simulink model "EZE4sLStEnCtrl"  (R2018b)
settings: Solver=FixedStepDiscrete  StartTime=0.0  StopTime=10.0  FixedStep=0.01  RelTol=1e-3
undefined symbols (not defined in the file or in its folder): data, SecRwLtStBkReclnEn_Clear, SecRwLtStBkReclnEn_Set, SecRwLtStFwdBkwdEn_Clear, SecRwLtStFwdBkwdEn_Set, SecRwLtStHdrstFwdBkwdEn_Clear, SecRwLtStHdrstFwdBkwdEn_Set, SecRwLtStHdrstUpwdDnwdEn_Clear, SecRwLtStHdrstUpwdDnwdEn_Set
libraries: simulink x1
settings Model: Creator=sn2xws  LastModifiedBy=sn55gm
settings DataIOCC: SaveFormat=StructureWithTime
settings OptimizationCC: DefaultParameterBehavior=Inlined  EnhancedBackFolding=on  PassReuseOutputArgsAs=Individual arguments  ZeroExternalMemoryAtStartup=off  ZeroInternalMemoryAtStartup=off  OptimizeBlockOrder=speed  DifferentSizesBufferReuse=on  OptimizationCustomize=off
settings DebuggingCC: ParameterTunabilityLossMsg=error
settings SFSimCC: MATLABDynamicMemAlloc=off
settings RTWCC: SystemTargetFile=autosar.tlc  GenCodeOnly=on  TemplateMakefile=ert_default_tmf  Description=AUTOSAR  GenerateReport=on  IncludeHyperlinkInReport=on  LaunchReport=on  GenerateTraceInfo=on  GenerateTraceReport=on  GenerateTraceReportSl=on  GenerateTraceReportSf=on  GenerateTraceReportEml=on  GenerateCodeMetricsReport=on
settings CodeAppCC: ForceParamTrailComments=on  IgnoreCustomStorageClasses=off  OperatorAnnotations=on  SimulinkDataObjDesc=on  SFDataObjDesc=on  InsertBlockDesc=on
settings STFCustomTargetCC: TargetLangStandard=C99 (ISO)  MultiwordLength=256  ParMdlRefBuildCompliant=on  CompOptLevelCompliant=on  IncludeMdlTerminateFcn=off  CombineOutputUpdateFcns=on  SuppressErrorStatus=on  ERTCustomFileBanners=on  SupportNonFinite=off  SupportComplex=off  SupportContinuousTime=off  SupportNonInlinedSFcns=off  RemoveResetFunc=on  MATLABClassNameForMDSCustomization=Simulink.SoftwareTarget.ERTCustomization  AutosarCompliant=on  UseToolchainInfoCompliant=on  LookupTableObjectStructAxisOrder=2,1,3,4,...  LUTObjectStructOrderEvenSpacing=Size,Table,Breakpoints  SystemTargetFile=autosar.tlc
settings ERTTargetCC: TargetLangStandard=C99 (ISO)  ConcurrentExecutionCompliant=off  IncludeMdlTerminateFcn=off  SuppressErrorStatus=on  SupportNonFinite=off  SupportComplex=off  ModelStepFunctionPrototypeControlCompliant=off  CPPClassGenCompliant=off  AutosarCompliant=on  LookupTableObjectStructAxisOrder=2,1,3,4,...  LUTObjectStructOrderEvenSpacing=Size,Table,Breakpoints  InlinedParameterPlacement=NonHierarchical  ERTCustomFileTemplate=example_file_process.tlc  ERTFilePackagingFormat=Compact

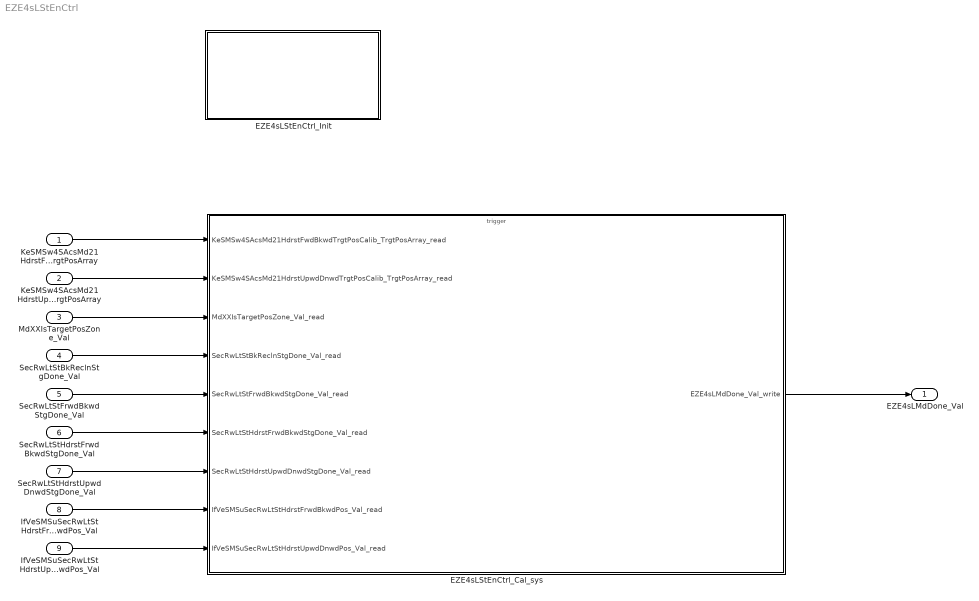
== system EZE4sLStEnCtrl ==
  KeSMSw4SAcsMd21HdrstFwdBkwdTrgtPosCalib_TrgtPosArray : Inport  Description=|  OutDataTypeStr=uint16  PortDimensions=3
      | 0:Pos
      | 1:Max
      | 2:Min
  KeSMSw4SAcsMd21HdrstUpwdDnwdTrgtPosCalib_TrgtPosArray : Inport  Description=|  Port=2  OutDataTypeStr=uint16  PortDimensions=3
      | 0:Pos
      | 1:Max
      | 2:Min
  MdXXIsTargetPosZone_Val : Inport  Port=3  OutDataTypeStr=uint32  PortDimensions=1
  SecRwLtStBkReclnStgDone_Val : Inport  Port=4  OutDataTypeStr=boolean  PortDimensions=1
  SecRwLtStFrwdBkwdStgDone_Val : Inport  Port=5  OutDataTypeStr=boolean  PortDimensions=1
  SecRwLtStHdrstFrwdBkwdStgDone_Val : Inport  Port=6  OutDataTypeStr=boolean  PortDimensions=1
  SecRwLtStHdrstUpwdDnwdStgDone_Val : Inport  Port=7  OutDataTypeStr=boolean  PortDimensions=1
  IfVeSMSuSecRwLtStHdrstFrwdBkwdPos_Val : Inport  Port=8  OutDataTypeStr=uint16  PortDimensions=1
  IfVeSMSuSecRwLtStHdrstUpwdDnwdPos_Val : Inport  Port=9  OutDataTypeStr=uint16  PortDimensions=1
  EZE4sLStEnCtrl_Cal_sys : Subsystem
  EZE4sLStEnCtrl_Init : Subsystem
  EZE4sLMdDone_Val : Outport  OutDataTypeStr=uint8  PortDimensions=1
  wires:
  KeSMSw4SAcsMd21HdrstFwdBkwdTrgtPosCalib_TrgtPosArray/1 -> EZE4sLStEnCtrl_Cal_sys/1(KeSMSw4SAcsMd21HdrstFwdBkwdTrgtPosCalib_TrgtPosArray_read)
  KeSMSw4SAcsMd21HdrstUpwdDnwdTrgtPosCalib_TrgtPosArray/1 -> EZE4sLStEnCtrl_Cal_sys/2(KeSMSw4SAcsMd21HdrstUpwdDnwdTrgtPosCalib_TrgtPosArray_read)
  MdXXIsTargetPosZone_Val/1 -> EZE4sLStEnCtrl_Cal_sys/3(MdXXIsTargetPosZone_Val_read)
  SecRwLtStBkReclnStgDone_Val/1 -> EZE4sLStEnCtrl_Cal_sys/4(SecRwLtStBkReclnStgDone_Val_read)
  SecRwLtStFrwdBkwdStgDone_Val/1 -> EZE4sLStEnCtrl_Cal_sys/5(SecRwLtStFrwdBkwdStgDone_Val_read)
  SecRwLtStHdrstFrwdBkwdStgDone_Val/1 -> EZE4sLStEnCtrl_Cal_sys/6(SecRwLtStHdrstFrwdBkwdStgDone_Val_read)
  SecRwLtStHdrstUpwdDnwdStgDone_Val/1 -> EZE4sLStEnCtrl_Cal_sys/7(SecRwLtStHdrstUpwdDnwdStgDone_Val_read)
  EZE4sLStEnCtrl_Cal_sys/1(EZE4sLMdDone_Val_write) -> EZE4sLMdDone_Val/1
  IfVeSMSuSecRwLtStHdrstFrwdBkwdPos_Val/1 -> EZE4sLStEnCtrl_Cal_sys/8(IfVeSMSuSecRwLtStHdrstFrwdBkwdPos_Val_read)
  IfVeSMSuSecRwLtStHdrstUpwdDnwdPos_Val/1 -> EZE4sLStEnCtrl_Cal_sys/9(IfVeSMSuSecRwLtStHdrstUpwdDnwdPos_Val_read)

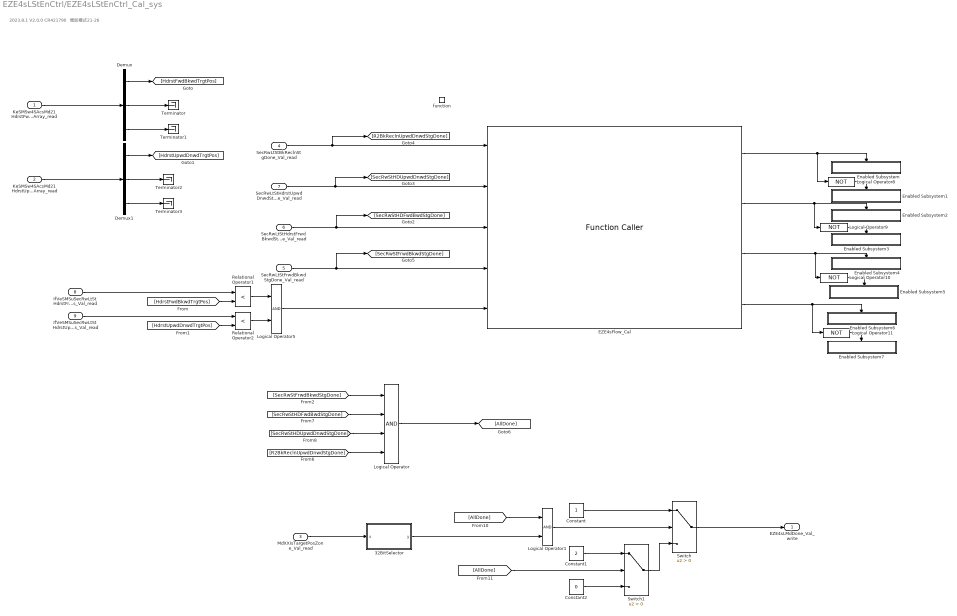
== system EZE4sLStEnCtrl/EZE4sLStEnCtrl_Cal_sys ==
  note: 2023.8.1 V2.0.0 CR421790 增加模式21-26
  KeSMSw4SAcsMd21HdrstFwdBkwdTrgtPosCalib_TrgtPosArray_read : Inport
  KeSMSw4SAcsMd21HdrstUpwdDnwdTrgtPosCalib_TrgtPosArray_read : Inport  Port=2
  MdXXIsTargetPosZone_Val_read : Inport  Port=3
  SecRwLtStBkReclnStgDone_Val_read : Inport  Port=4
  SecRwLtStFrwdBkwdStgDone_Val_read : Inport  Port=5
  SecRwLtStHdrstFrwdBkwdStgDone_Val_read : Inport  Port=6
  SecRwLtStHdrstUpwdDnwdStgDone_Val_read : Inport  Port=7
  IfVeSMSuSecRwLtStHdrstFrwdBkwdPos_Val_read : Inport  Port=8
  IfVeSMSuSecRwLtStHdrstUpwdDnwdPos_Val_read : Inport  Port=9
  function : TriggerPort  TriggerType=function-call  IsSimulinkFunction=on  FunctionName=EZE4sLStEnCtrl_Cal  VariantControl=(inherit)
  32BitSelector : Subsystem  mask(32 Bit Selector){BitNum=20}
      mask prompts: BitNum "Select Bit Number"
      mask help: Allows selection of a particular bit (0-31) out of a packed word up to 32 bits long. Output will be true if the bit number selected via the mask parameter is equal to one.
      mask TypeOptions BitNum: 0 | 1 | 2 | 3 | 4 | 5 | 6 | 7 | 8 | 9 | 10 | 11 | 12 | 13 | 14 | 15 | 16 | 17 | 18 | 19 | 20 | 21 | 22 | 23 | 24 | 25 | 26 | 27 | 28 | 29 | 30 | 31
      mask Display:
      | text(0.5, 0.8,'BIT','horizontalAlignment','center')
      | text(0.5, 0.5,'SELECTOR','horizontalAlignment','center')
      | text(0.5, 0.2,['-- Bit ',char(get_param(gcb,'BitNum')),' --'],'horizontalAlignment','center')
  Constant : Constant  OutDataTypeStr=uint8
  Constant1 : Constant  Value=2  OutDataTypeStr=uint8
  Constant2 : Constant  Value=0  OutDataTypeStr=uint8
  Demux : Demux  Outputs=3
  Demux1 : Demux  Outputs=3
  EZE4sFlow_Cal : FunctionCaller  FunctionPrototype=[BkReclnEn,HdrstUpwdEn,HdrstFrwdEn,SecRwStFrwdBkwdEn] = EZE4sFlow_Cal(BkReclnStgDone,HdrstUpwdDnwdStgDone,HdrstFrwdBkwdStgDone,SecRwStFrwdBkwdStgDone,Chkhdflg)  InputArgumentSpecifications=boolean(true), boolean(true), boolean(true), boolean(true), boolean(true)  OutputArgumentSpecifications=boolean(true), boolean(true), boolean(true), boolean(true)
  Enabled Subsystem : Subsystem  TreatAsAtomicUnit=on
  Enabled Subsystem1 : Subsystem  TreatAsAtomicUnit=on
  Enabled Subsystem2 : Subsystem  TreatAsAtomicUnit=on
  Enabled Subsystem3 : Subsystem  TreatAsAtomicUnit=on
  Enabled Subsystem4 : Subsystem  TreatAsAtomicUnit=on
  Enabled Subsystem5 : Subsystem  TreatAsAtomicUnit=on
  Enabled Subsystem6 : Subsystem  TreatAsAtomicUnit=on
  Enabled Subsystem7 : Subsystem  TreatAsAtomicUnit=on
  Logical Operator : Logic  Inputs=4  AllPortsSameDT=off  OutDataTypeStr=boolean
  Logical Operator1 : Logic  AllPortsSameDT=off  OutDataTypeStr=boolean
  Logical Operator{8..11} (4 alike) : Logic  Operator=NOT  AllPortsSameDT=off  OutDataTypeStr=boolean
  Logical Operator5 : Logic  AllPortsSameDT=off  OutDataTypeStr=boolean
  Relational Operator1 : RelationalOperator  Operator=<  OutDataTypeStr=boolean  RndMeth=Simplest
  Relational Operator2 : RelationalOperator  Operator=<  OutDataTypeStr=boolean  RndMeth=Simplest
  Switch : Switch  Criteria=u2 > Threshold
  Switch1 : Switch  Criteria=u2 > Threshold
  Terminator{,1..3} (4 alike) : Terminator
  EZE4sLMdDone_Val_write : Outport
      settings: EnsureOutportIsVirtual=on
  wires:
  Relational Operator1/1 -> Logical Operator5/1
  Logical Operator5/1 -> EZE4sFlow_Cal/5
  Relational Operator2/1 -> Logical Operator5/2
  SecRwLtStBkReclnStgDone_Val_read/1 -> [R2BkReclnUpwdDnwdStgDone], EZE4sFlow_Cal/1
  SecRwLtStHdrstUpwdDnwdStgDone_Val_read/1 -> [SecRwStHDUpwdDnwdStgDone], EZE4sFlow_Cal/2
  SecRwLtStFrwdBkwdStgDone_Val_read/1 -> [SecRwStFrwdBkwdStgDone], EZE4sFlow_Cal/4
  SecRwLtStHdrstFrwdBkwdStgDone_Val_read/1 -> [SecRwStHDFwdBwdStgDone], EZE4sFlow_Cal/3
  IfVeSMSuSecRwLtStHdrstFrwdBkwdPos_Val_read/1 -> Relational Operator1/1
  IfVeSMSuSecRwLtStHdrstUpwdDnwdPos_Val_read/1 -> Relational Operator2/1
  KeSMSw4SAcsMd21HdrstFwdBkwdTrgtPosCalib_TrgtPosArray_read/1 -> Demux/1
  Demux/1 -> [HdrstFwdBkwdTrgtPos]
  KeSMSw4SAcsMd21HdrstUpwdDnwdTrgtPosCalib_TrgtPosArray_read/1 -> Demux1/1
  Demux1/1 -> [HdrstUpwdDnwdTrgtPos]
  Demux/2 -> Terminator/1
  Demux/3 -> Terminator1/1
  Demux1/2 -> Terminator2/1
  Demux1/3 -> Terminator3/1
  [HdrstFwdBkwdTrgtPos] -> Relational Operator1/2
  [HdrstUpwdDnwdTrgtPos] -> Relational Operator2/2
  [SecRwStHDUpwdDnwdStgDone] -> Logical Operator/3
  [SecRwStHDFwdBwdStgDone] -> Logical Operator/2
  [R2BkReclnUpwdDnwdStgDone] -> Logical Operator/4
  [SecRwStFrwdBkwdStgDone] -> Logical Operator/1
  Constant1/1 -> Switch1/1
  Constant/1 -> Switch/1
  Switch1/1 -> Switch/3
  Logical Operator1/1 -> Switch/2
  [AllDone] -> Logical Operator1/1
  32BitSelector/1(y) -> Logical Operator1/2
  Switch/1 -> EZE4sLMdDone_Val_write/1
  [AllDone] -> Switch1/2
  MdXXIsTargetPosZone_Val_read/1 -> 32BitSelector/1(x)
  Constant2/1 -> Switch1/3
  Logical Operator/1 -> [AllDone]
  EZE4sFlow_Cal/2 -> Logical Operator9/1, Enabled Subsystem2/Enable
  Logical Operator10/1 -> Enabled Subsystem5/Enable
  Logical Operator8/1 -> Enabled Subsystem1/Enable
  EZE4sFlow_Cal/3 -> Logical Operator10/1, Enabled Subsystem4/Enable
  EZE4sFlow_Cal/1 -> Logical Operator8/1, Enabled Subsystem/Enable
  Logical Operator9/1 -> Enabled Subsystem3/Enable
  Logical Operator11/1 -> Enabled Subsystem7/Enable
  EZE4sFlow_Cal/4 -> Logical Operator11/1, Enabled Subsystem6/Enable

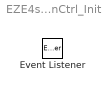
== system EZE4sLStEnCtrl/EZE4sLStEnCtrl_Init ==
  Event Listener : EventListener  EventName=reset

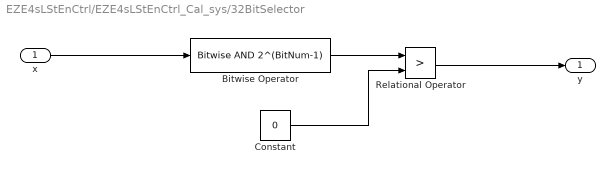
== system EZE4sLStEnCtrl/EZE4sLStEnCtrl_Cal_sys/32BitSelector ==
  x : Inport
  Bitwise Operator : simulink/Logic and Bit Operations/Bitwise Operator  logicop=AND  UseBitMask=on  BitMask=2^(BitNum-1)  BitMaskRealWorld=Stored Integer
  Constant : Constant  Value=0  OutDataTypeStr=uint32
  Relational Operator : RelationalOperator  Operator=>  OutDataTypeStr=boolean  RndMeth=Simplest
  y : Outport
  wires:
  Relational Operator/1 -> y/1
  Constant/1 -> Relational Operator/2
  x/1 -> Bitwise Operator/1
  Bitwise Operator/1 -> Relational Operator/1

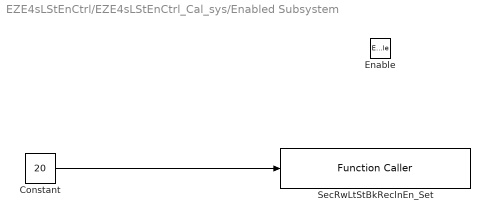
== system EZE4sLStEnCtrl/EZE4sLStEnCtrl_Cal_sys/Enabled Subsystem ==
  Enable : EnablePort
  Constant : Constant  Value=20  OutDataTypeStr=uint8
  SecRwLtStBkReclnEn_Set : FunctionCaller  FunctionPrototype=SecRwLtStBkReclnEn_Set(data)  InputArgumentSpecifications=uint8(1)
  wires:
  Constant/1 -> SecRwLtStBkReclnEn_Set/1

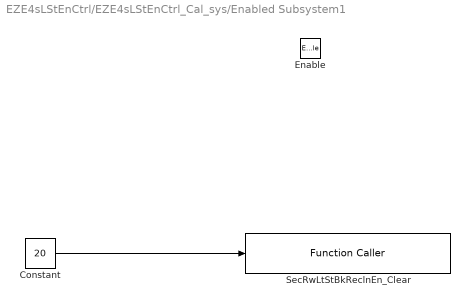
== system EZE4sLStEnCtrl/EZE4sLStEnCtrl_Cal_sys/Enabled Subsystem1 ==
  Enable : EnablePort
  Constant : Constant  Value=20  OutDataTypeStr=uint8
  SecRwLtStBkReclnEn_Clear : FunctionCaller  FunctionPrototype=SecRwLtStBkReclnEn_Clear(data)  InputArgumentSpecifications=uint8(1)
  wires:
  Constant/1 -> SecRwLtStBkReclnEn_Clear/1

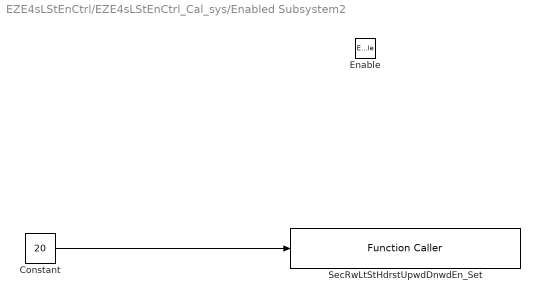
== system EZE4sLStEnCtrl/EZE4sLStEnCtrl_Cal_sys/Enabled Subsystem2 ==
  Enable : EnablePort
  Constant : Constant  Value=20  OutDataTypeStr=uint8
  SecRwLtStHdrstUpwdDnwdEn_Set : FunctionCaller  FunctionPrototype=SecRwLtStHdrstUpwdDnwdEn_Set(data)  InputArgumentSpecifications=uint8(1)
  wires:
  Constant/1 -> SecRwLtStHdrstUpwdDnwdEn_Set/1

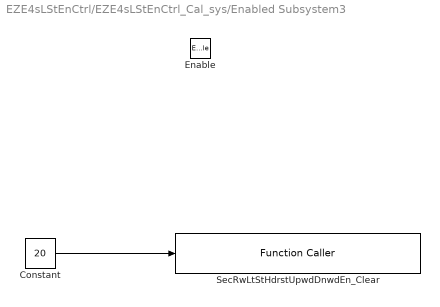
== system EZE4sLStEnCtrl/EZE4sLStEnCtrl_Cal_sys/Enabled Subsystem3 ==
  Enable : EnablePort
  Constant : Constant  Value=20  OutDataTypeStr=uint8
  SecRwLtStHdrstUpwdDnwdEn_Clear : FunctionCaller  FunctionPrototype=SecRwLtStHdrstUpwdDnwdEn_Clear(data)  InputArgumentSpecifications=uint8(1)
  wires:
  Constant/1 -> SecRwLtStHdrstUpwdDnwdEn_Clear/1

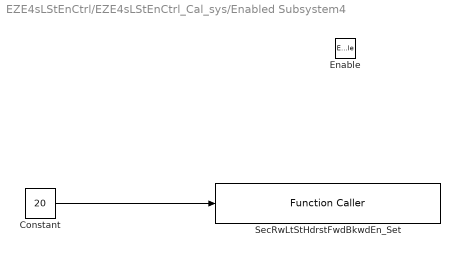
== system EZE4sLStEnCtrl/EZE4sLStEnCtrl_Cal_sys/Enabled Subsystem4 ==
  Enable : EnablePort
  Constant : Constant  Value=20  OutDataTypeStr=uint8
  SecRwLtStHdrstFwdBkwdEn_Set : FunctionCaller  FunctionPrototype=SecRwLtStHdrstFwdBkwdEn_Set(data)  InputArgumentSpecifications=uint8(1)
  wires:
  Constant/1 -> SecRwLtStHdrstFwdBkwdEn_Set/1

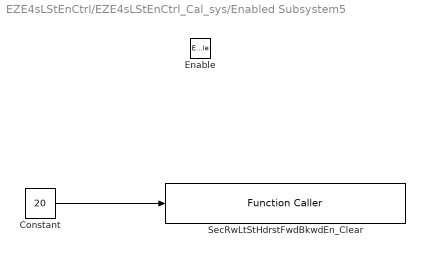
== system EZE4sLStEnCtrl/EZE4sLStEnCtrl_Cal_sys/Enabled Subsystem5 ==
  Enable : EnablePort
  Constant : Constant  Value=20  OutDataTypeStr=uint8
  SecRwLtStHdrstFwdBkwdEn_Clear : FunctionCaller  FunctionPrototype=SecRwLtStHdrstFwdBkwdEn_Clear(data)  InputArgumentSpecifications=uint8(1)
  wires:
  Constant/1 -> SecRwLtStHdrstFwdBkwdEn_Clear/1

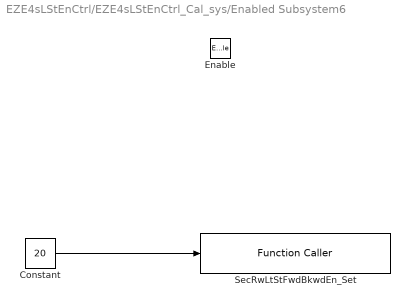
== system EZE4sLStEnCtrl/EZE4sLStEnCtrl_Cal_sys/Enabled Subsystem6 ==
  Enable : EnablePort
  Constant : Constant  Value=20  OutDataTypeStr=uint8
  SecRwLtStFwdBkwdEn_Set : FunctionCaller  FunctionPrototype=SecRwLtStFwdBkwdEn_Set(data)  InputArgumentSpecifications=uint8(1)
  wires:
  Constant/1 -> SecRwLtStFwdBkwdEn_Set/1

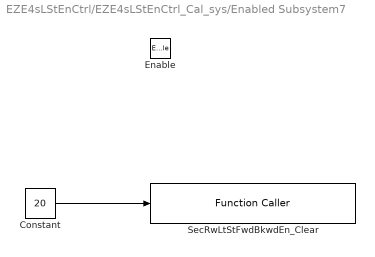
== system EZE4sLStEnCtrl/EZE4sLStEnCtrl_Cal_sys/Enabled Subsystem7 ==
  Enable : EnablePort
  Constant : Constant  Value=20  OutDataTypeStr=uint8
  SecRwLtStFwdBkwdEn_Clear : FunctionCaller  FunctionPrototype=SecRwLtStFwdBkwdEn_Clear(data)  InputArgumentSpecifications=uint8(1)
  wires:
  Constant/1 -> SecRwLtStFwdBkwdEn_Clear/1
